simulink model "mcb_pmsm_foc_abs_current_loop_mex"  (R2024a)
settings: Solver=FixedStepAuto  StartTime=0.0  StopTime=2  FixedStep=1e-6  RelTol=1e-3
undefined symbols (not defined in the file): motor
libraries: simulink_extras x4, spsDCVoltageSourceLib x1, eePwmGeneratorTwoLevel x1, spsUniversalBridgeLib x1, spsPermanentMagnetSynchronousMachineLib x1, spsThreePhaseVIMeasurementLib x1, sps_lib x1
settings Model: Creator=dark  LastModifiedBy=dark

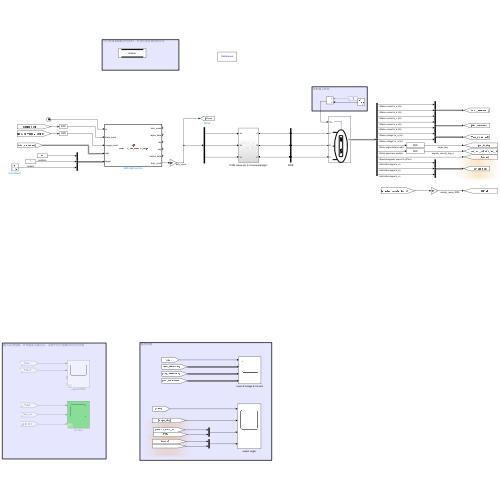
[thumbnail: Simulink's stored preview of the top-level diagram]
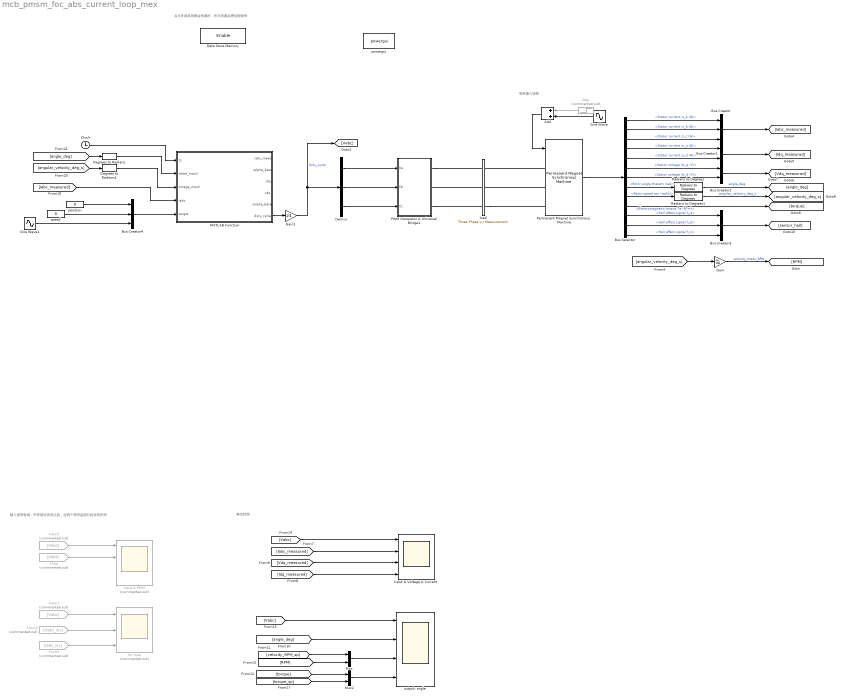
== system mcb_pmsm_foc_abs_current_loop_mex ==
  note: 电机输入转矩
  note: 当与外部系统联合仿真时，作为仿真启停控制信号
  note: 输出检测
  note: 输入信号检测：开环验证完成之后，这两个信号监测已经没有作用
  Add : Sum
  Bus Creator : BusCreator  Inputs=3
  Bus Creator1 : BusCreator  Inputs=2
  Bus Creator2 : BusCreator  Inputs=2
  Bus Creator3 : BusCreator  Inputs=3
  Bus Creator4 : BusCreator  Inputs=3
  Bus Selector : BusSelector  OutputSignals=Stator current is_a (A),Stator current is_b (A),Stator current is_c (A),Stator current is_q (A),Stator current is_d (A),Stator voltage Vs_q (V),Stator voltage Vs_d (V),Rotor angle thetam (rad),Rotor speed wm (rad/s),Electromagnetic torque Te (N*m),Hall effect signal h_a,Hall effect signal h_b,Hall effect signal h_c
  Clock : Clock
  Data Store Memory : DataStoreMemory  DataStoreName=Enable  WriteAfterWriteMsg=warning  InitialValue=1  ShowAdditionalParam=off  OutDataTypeStr=boolean
  Degrees to Radians : simulink_extras/Transformations/Degrees to Radians
  Degrees to Radians1 : simulink_extras/Transformations/Degrees to Radians
  Demux : Demux  Outputs=3
  From : From  Commented=on  GotoTag=PWM
  From1 : From  Commented=on  GotoTag=Vabc
  From2 : From  Commented=on  GotoTag=Vabc_inv  TagVisibility=global
  From5 : From  Commented=on  GotoTag=Vabc
  From6 : From  Commented=on  GotoTag=Iabc_inv  TagVisibility=global
  Gain : Gain  Gain=60 / 360
  Gain1 : Gain  Gain=24
  Input & PWM : Scope  Commented=on  NumInputPorts=4
  Input & Voltage & Current : Scope  NumInputPorts=4
  Inv Sine : Scope  Commented=on  NumInputPorts=3
  MATLAB Function : MATLAB Function  TreatAsAtomicUnit=on
  Mux : Mux  Inputs=2
  Mux2 : Mux  Inputs=2
  PWM Generator & Universal Bridge1 : Subsystem
  Permanent Magnet Synchronous Machine : spsPermanentMagnetSynchronousMachineLib/Permanent Magnet Synchronous Machine  NbPhases=3  FluxDistribution=Sinusoidal  RotorType=Salient-pole  MechanicalLoad=Torque Tm  PresetModel=No  ShowDetailedParameters=on  MeasurementBus=off  Resistance=motor.phase_resistance  Inductance=8.5e-3  dqInductances=[motor.phase_inductance, motor.phase_inductance]  La=0.000395  MachineConstant=Torque Constant (N.m / A_peak)  Flux=0.0078901  VoltageCst=7.1555  TorqueCst=motor.torque_constant  Flat=120  Mechanical=[motor.inertia motor.friction_damping_factor motor.pole_pairs 0]  PolePairs=4  InitialConditions=[0,0, 0,0]  InitialConditions5ph=[0 0 0 0 0 0]  RefAngle=Aligned with phase A axis (original Park)  IterativeDiscreteModel=Trapezoidal non iterative  TsBlock=-1  TsPowergui=0
  Radians to Degrees : simulink_extras/Transformations/Radians to Degrees
  Radians to Degrees1 : simulink_extras/Transformations/Radians to Degrees
  Sine Wave : Sin  Amplitude=0.45  Frequency=2*pi*10  SampleTime=0
  Sine Wave1 : Sin  Amplitude=0.5  Frequency=2*pi*10  SampleTime=0
  Step : Step  Commented=on  Time=0.2  After=0.05  SampleTime=0
  load : spsThreePhaseVIMeasurementLib/Three-Phase V-I Measurement  VoltageMeasurement=phase-to-phase  SetLabelV=on  LabelV=Vabc_inv  Vpu=off  VpuLL=off  CurrentMeasurement=yes  SetLabelI=on  LabelI=Iabc_inv  Ipu=off  Pbase=1e3  Vbase=380  OutputType=Magnitude  PhasorSimulation=off  PSBequivalent=0
  output: angle : Scope  NumInputPorts=4
  position : Constant  Value=0
  powergui : sps_lib/powergui  Priority=1  SimulationMode=Continuous  SampleTime=50e-6  frequency=60  Iterations=50  frequencyindice=0  Pbase=100e6  ErrMax=1e-4  UnitsV=kV  UnitsW=MW  buscounter=0  FunctionMessages=off  echomessages=off  EnableUseOfTLC=off  CurrentSourceSwitches=off  DisableSnubberDevices=off  DisableRonSwitches=off  DisableVfSwitches=off  DisplayEquations=off  AutomaticDiscreteSolvers=off  SolverType=Tustin/Backward Euler (TBE)  Interpol=off  ExternalGateDelay=off  methode=off  Ts=100  x0status=blocks  SPID=on  SwTol=0  HookPort=off  NonlinearTolerance=1e-4  nMaxIteration=100  ContinueOnMaxIteration=off  RestoreLinks=warning  ResistiveCurrentMeasurement=off  Frange=[0:2:500]  Ylog=off  Xlog=on  ShowGrid=off  save=off  variable=ZData  structure=0  ZoomFFT=off  StartTime=0.0  cycles=1  DisplayStyle=1  fundamental=60  FreqAxis=off  MaxFrequency=1000  frequencyindicesteady=1  RmsSteady=1  display=off
  speed : Constant  Value=0
  wires:
  Permanent Magnet Synchronous Machine/1 -> Bus Selector/1
  Bus Selector/1 -> Bus Creator/1  "<Stator current is_a (A)>"
  Bus Selector/2 -> Bus Creator/2  "<Stator current is_b (A)>"
  Bus Selector/3 -> Bus Creator/3  "<Stator current is_c (A)>"
  From1/1 -> Inv Sine/1
  From6/1 -> Inv Sine/3
  From2/1 -> Inv Sine/2
  Bus Creator/1 -> [Iabc_measured]
  Bus Selector/4 -> Bus Creator1/1  "<Stator current is_q (A)>"
  Bus Selector/5 -> Bus Creator1/2  "<Stator current is_d (A)>"
  Bus Creator1/1 -> [Idq_measured]
  Bus Selector/10 -> [torque]  "<Electromagnetic torque Te (N*m)>"
  Bus Selector/8 -> Radians to Degrees/1  "<Rotor angle thetam (rad)>"
  Bus Selector/9 -> Radians to Degrees1/1  "<Rotor speed wm (rad/s)>"
  Bus Selector/6 -> Bus Creator2/1  "<Stator voltage Vs_q (V)>"
  Bus Selector/7 -> Bus Creator2/2  "<Stator voltage Vs_d (V)>"
  Bus Creator2/1 -> [Vdq_measured]
  Bus Creator3/1 -> [sensor_hall]
  Bus Selector/11 -> Bus Creator3/1  "<Hall effect signal h_a>"
  Bus Selector/12 -> Bus Creator3/2  "<Hall effect signal h_b>"
  Bus Selector/13 -> Bus Creator3/3  "<Hall effect signal h_c>"
  [Idq_measured] -> Input & Voltage & Current/4
  [Vdq_measured] -> Input & Voltage & Current/3
  [Iabc_measured] -> Input & Voltage & Current/2
  [Vabc] -> Input & Voltage & Current/1
  Radians to Degrees/1 -> [angle_deg]  "angle_deg"
  Radians to Degrees1/1 -> [angular_velocity_deg_s]  "angular_velocity_deg_s"
  [angle_deg] -> output: angle/2
  [Vabc] -> output: angle/1
  From5/1 -> Input & PWM/1
  From/1 -> Input & PWM/2
  Add/1 -> Permanent Magnet Synchronous Machine/1
  Step/1 -> Add/1
  Sine Wave/1 -> Add/2
  [angular_velocity_deg_s] -> Gain/1
  Gain/1 -> [RPM]  "velocity_meas_RPM"
  Mux/1 -> output: angle/3
  [velocity_RPM_sp] -> Mux/1
  [RPM] -> Mux/2
  Sine Wave1/1 -> Bus Creator4/3
  Mux2/1 -> output: angle/4
  [torque] -> Mux2/1
  [torque_sp] -> Mux2/2
  speed/1 -> Bus Creator4/2
  position/1 -> Bus Creator4/1
  Bus Creator4/1 -> MATLAB Function/5(target)
  [Iabc_measured] -> MATLAB Function/4(iabc)
  [angular_velocity_deg_s] -> Degrees to Radians1/1
  [angle_deg] -> Degrees to Radians/1
  Clock/1 -> MATLAB Function/1(ts)
  MATLAB Function/6(duty_cycle) -> Gain1/1
  Degrees to Radians/1 -> MATLAB Function/2(theta_mach)
  Degrees to Radians1/1 -> MATLAB Function/3(omega_mach)
  Demux/1 -> PWM Generator & Universal Bridge1/1(Va)
  Demux/2 -> PWM Generator & Universal Bridge1/2(Vb)
  Demux/3 -> PWM Generator & Universal Bridge1/3(Vc)
  Gain1/1 -> Demux/1, [Vabc]  "duty_cycle"
  connections:
  load/RConn3 -- Permanent Magnet Synchronous Machine/LConn3
  Permanent Magnet Synchronous Machine/LConn1 -- load/RConn1
  Permanent Magnet Synchronous Machine/LConn2 -- load/RConn2
  PWM Generator & Universal Bridge1/RConn1 -- load/LConn1
  load/LConn2 -- PWM Generator & Universal Bridge1/RConn2
  PWM Generator & Universal Bridge1/RConn3 -- load/LConn3

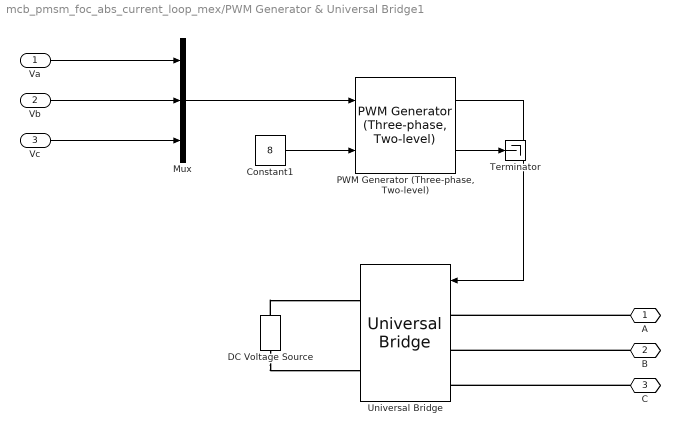
== system mcb_pmsm_foc_abs_current_loop_mex/PWM Generator & Universal Bridge1 ==
  Va : Inport
  Vb : Inport  Port=2
  Vc : Inport  Port=3
  Constant1 : Constant  Value=8
  DC Voltage Source : spsDCVoltageSourceLib/DC Voltage Source  Amplitude=motor.voltage  Measurements=Voltage
  Mux : Mux  Inputs=3
  "PWM Generator (Three-phase, Two-level)" : eePwmGeneratorTwoLevel/PWM Generator (Three-phase, Two-level)  PWMMode=Continuous PWM (CPWM)  CPWMMode=SPWM: sinusoidal PWM  DPWMMode=60 DPWM: 60 degree discontinuous PWM  fsw=PWM.frequency  Ts=1e-6
      settings: LibrarySourceBlock=|
      | ee_sl_lib/Pulse Width
      | Modulation/PWM Generator
      | (Three-phase, Two-level)
  Terminator : Terminator
  Universal Bridge : spsUniversalBridgeLib/Universal Bridge  Arms=3  SnubberResistance=1e6  SnubberCapacitance=inf  Device=MOSFET / Diodes  Ron=1e-3  Lon=0  ForwardVoltages="[  0  0  ]"  ForwardVoltage=0  GTOparameters=[ 10e-6 , 20e-6 ]  IGBTparameters=[ 1e-6 , 2e-6 ]  Measurements=All voltages and currents  Measurements_2=None  converterType=Rectifier
  A : PMIOPort  Side=Right
  B : PMIOPort  Port=2  Side=Right
  C : PMIOPort  Port=3  Side=Right
  wires:
  "PWM Generator (Three-phase, Two-level)"/1 -> Universal Bridge/1
  Constant1/1 -> "PWM Generator (Three-phase, Two-level)"/2
  "PWM Generator (Three-phase, Two-level)"/2 -> Terminator/1
  Mux/1 -> "PWM Generator (Three-phase, Two-level)"/1
  Vc/1 -> Mux/3
  Vb/1 -> Mux/2
  Va/1 -> Mux/1
  connections:
  B/RConn1 -- Universal Bridge/LConn2
  DC Voltage Source/LConn1 -- Universal Bridge/RConn2
  DC Voltage Source/RConn1 -- Universal Bridge/RConn1
  C/RConn1 -- Universal Bridge/LConn3
  A/RConn1 -- Universal Bridge/LConn1

== matlab function mcb_pmsm_foc_abs_current_loop_mex/MATLAB Function ==
  data: ts input; iabc_meas output; theta_mach input; omega_mach input; iabc input; ialpha_beta output; idq output; vdq output; valpha_beta output; duty_cycle output; target input
function [iabc_meas,ialpha_beta,idq,vdq,valpha_beta, duty_cycle] = picadrive_foc_current_loop(ts, theta_mach, omega_mach, iabc, target)
    coder.extrinsic('mex_picadrive_bldc_foc');
    
    iabc_meas = zeros(3,1);
    ialpha_beta = zeros(2,1);
    idq = zeros(2, 1);
    vdq = zeros(2, 1);
    valpha_beta = zeros(2, 1);
    duty_cycle = zeros(3, 1);

    [iabc_meas, ialpha_beta, idq, vdq, valpha_beta, duty_cycle] = mex_picadrive_bldc_foc(ts, theta_mach, omega_mach, iabc, target);
